simulink model "Energy2021b"  (R2021b)
settings: Solver=ode1  StartTime=0.0  StopTime=955800  FixedStep=1  RelTol=1e-3
(part 1 of 3)
settings Model: Creator=YYH  LastModifiedBy=10537
settings DebuggingCC: UnconnectedInputMsg=none  UnconnectedOutputMsg=none  UnconnectedLineMsg=none
settings ModelReferenceCC: EnableRefExpFcnMdlSchedulingChecks=off
settings RTWCC: GPUComputeCapability=5.0  DLArmComputeVersion=20.02.1

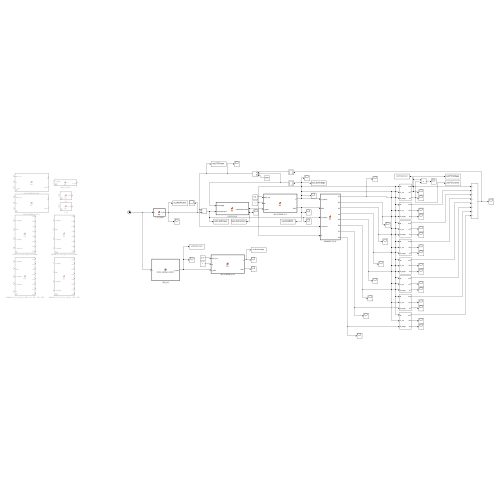
[thumbnail: Simulink's stored preview of the top-level diagram]
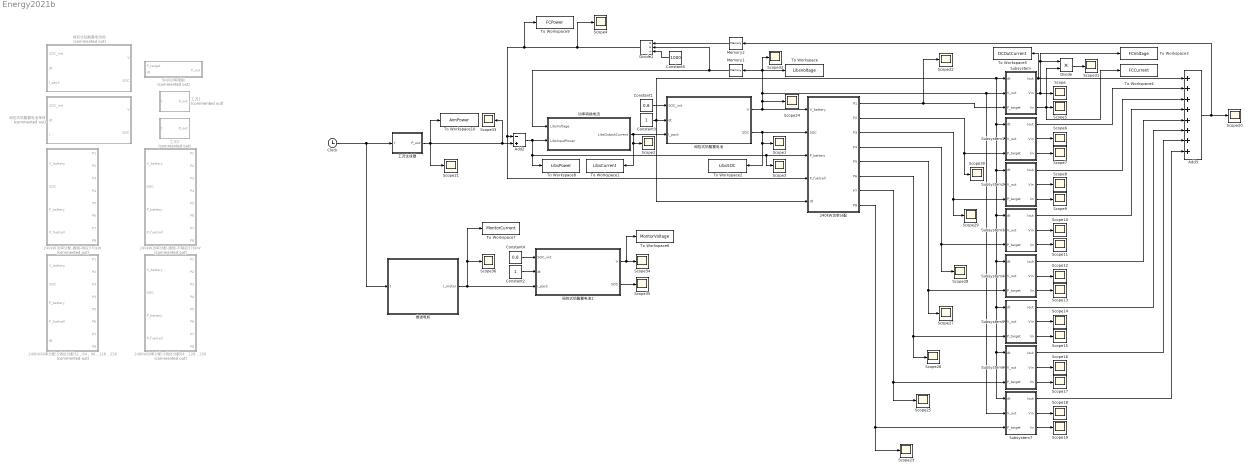
== system Energy2021b ==
  240kW功率分配 : MATLAB Function  TreatAsAtomicUnit=on
  240kW功率分配-3挡位分配64，128，256 : MATLAB Function  Commented=on  TreatAsAtomicUnit=on
  240kW功率分配-5挡位分配32，64，96，128，256 : MATLAB Function  Commented=on  TreatAsAtomicUnit=on
  240kW功率分配-跟随-不响应370kW : MATLAB Function  Commented=on  TreatAsAtomicUnit=on
  240kW功率分配-跟随-响应370kW : MATLAB Function  Commented=on  TreatAsAtomicUnit=on
  5kW功率限制 : MATLAB Function  Commented=on  TreatAsAtomicUnit=on
  Add2 : Sum  Inputs=-+
  Add3 : Sum  Inputs=++++++++
  Clock : Clock
  Constant1 : Constant  Value=0.8
  Constant2 : Constant
  Constant3 : Constant
  Constant4 : Constant  Value=0.8
  Constant5 : Constant  Value=1000
  Divide : Product  Inputs=**
  Divide1 : Product  Inputs=**/
  Memory1 : Memory  InitialCondition=487.0548
  Memory2 : Memory
  Scope{,1..36} (37 alike) : Scope
  Subsystem : Subsystem
  Subsystem1 : Subsystem
  Subsystem2 : Subsystem
  Subsystem3 : Subsystem
  Subsystem4 : Subsystem
  Subsystem5 : Subsystem
  Subsystem6 : Subsystem
  Subsystem7 : Subsystem
  To Workspace : ToWorkspace  VariableName=LibsVoltage  SaveFormat=Structure With Time  SampleTime=-1
  To Workspace1 : ToWorkspace  VariableName=LibsCurrent  SaveFormat=Structure With Time  SampleTime=-1
  To Workspace10 : ToWorkspace  VariableName=AimPower  SaveFormat=Structure With Time  SampleTime=-1
  To Workspace2 : ToWorkspace  VariableName=LibsSOC  SaveFormat=Structure With Time  SampleTime=-1
  To Workspace3 : ToWorkspace  VariableName=FCVoltage  SaveFormat=Structure With Time  SampleTime=-1
  To Workspace4 : ToWorkspace  VariableName=FCCurrent  SaveFormat=Structure With Time  SampleTime=-1
  To Workspace5 : ToWorkspace  VariableName=DCOutCurrent  SaveFormat=Structure With Time  SampleTime=-1
  To Workspace6 : ToWorkspace  VariableName=MontorVoltage  SaveFormat=Structure With Time  SampleTime=-1
  To Workspace7 : ToWorkspace  VariableName=MontorCurrent  SaveFormat=Structure With Time  SampleTime=-1
  To Workspace8 : ToWorkspace  VariableName=LibsPower  SaveFormat=Structure With Time  SampleTime=-1
  To Workspace9 : ToWorkspace  VariableName=FCPower  SaveFormat=Structure With Time  SampleTime=-1
  功率转换电流 : MATLAB Function  TreatAsAtomicUnit=on
  工况1 : MATLAB Function  Commented=on  TreatAsAtomicUnit=on
  工况2 : MATLAB Function  Commented=on  TreatAsAtomicUnit=on
  工况生成器 : MATLAB Function  TreatAsAtomicUnit=on
  推进电机 : MATLAB Function  TreatAsAtomicUnit=on
  阀控式铅酸蓄电池 : MATLAB Function  TreatAsAtomicUnit=on
  阀控式铅酸蓄电池1 : MATLAB Function  TreatAsAtomicUnit=on
  阀控式铅酸蓄电池单体 : MATLAB Function  Commented=on  TreatAsAtomicUnit=on
  阀控式铅酸蓄电池组 : MATLAB Function  Commented=on  TreatAsAtomicUnit=on
  wires:
  功率转换电流/1(LibsOutputCurrent) -> 阀控式铅酸蓄电池/3(I_pack), To Workspace1/1, Scope2/1
  Memory1/1 -> Divide1/2, 功率转换电流/1(LibsVoltage)
  阀控式铅酸蓄电池/2(SOC) -> To Workspace2/1, Scope1/1, 240kW功率分配/2(SOC)
  Constant1/1 -> 阀控式铅酸蓄电池/1(SOC_init)
  Memory2/1 -> Divide1/1
  Divide1/1 -> Scope4/1, To Workspace9/1, 240kW功率分配/4(P_fuelcell), Add2/1
  Constant5/1 -> Divide1/3
  240kW功率分配/1(P1) -> Scope22/1, Subsystem/3(P_target)
  240kW功率分配/2(P2) -> Scope30/1, Subsystem1/3(P_target)
  240kW功率分配/3(P3) -> Subsystem2/3(P_target), Scope29/1
  240kW功率分配/4(P4) -> Subsystem3/3(P_target), Scope28/1
  240kW功率分配/5(P5) -> Scope27/1, Subsystem4/3(P_target)
  240kW功率分配/8(P8) -> Subsystem7/3(P_target), Scope23/1
  240kW功率分配/7(P7) -> Subsystem6/3(P_target), Scope25/1
  Subsystem/1(Iout) -> To Workspace5/1, Add3/1
  Subsystem1/1(Iout) -> Add3/2
  Subsystem2/1(Iout) -> Add3/3
  Subsystem7/1(Iout) -> Add3/8
  Subsystem6/1(Iout) -> Add3/7
  Subsystem5/1(Iout) -> Add3/6
  Subsystem4/1(Iout) -> Add3/5
  Subsystem3/1(Iout) -> Add3/4
  Subsystem/2(Vin) -> To Workspace3/1, Divide/1, Scope/1
  Subsystem/3(Iin) -> Scope5/1, To Workspace4/1, Divide/2
  Subsystem1/3(Iin) -> Scope7/1
  Subsystem1/2(Vin) -> Scope6/1
  Subsystem2/2(Vin) -> Scope8/1
  Subsystem2/3(Iin) -> Scope9/1
  Subsystem3/2(Vin) -> Scope10/1
  Subsystem3/3(Iin) -> Scope11/1
  Subsystem4/2(Vin) -> Scope12/1
  Subsystem4/3(Iin) -> Scope13/1
  Subsystem7/3(Iin) -> Scope19/1
  Subsystem7/2(Vin) -> Scope18/1
  Subsystem6/3(Iin) -> Scope17/1
  Subsystem6/2(Vin) -> Scope16/1
  Subsystem5/3(Iin) -> Scope15/1
  Subsystem5/2(Vin) -> Scope14/1
  Add3/1 -> Memory2/1, Scope20/1
  Add2/1 -> To Workspace8/1, 240kW功率分配/3(P_battery), Scope3/1, 功率转换电流/2(LibsInputPower)
  阀控式铅酸蓄电池/1(V) -> Scope24/1, Subsystem/2(V_out), Subsystem1/2(V_out), Subsystem2/2(V_out), Subsystem3/2(V_out), Subsystem4/2(V_out), Subsystem5/2(V_out), Subsystem7/2(V_out), Subsystem6/2(V_out), Scope32/1, Memory1/1, To Workspace/1, 240kW功率分配/1(V_battery)
  240kW功率分配/6(P6) -> Subsystem5/3(P_target), Scope26/1
  Divide/1 -> Scope31/1
  Constant3/1 -> 240kW功率分配/5(dt), 阀控式铅酸蓄电池/2(dt), Subsystem1/1(dt), Subsystem2/1(dt), Subsystem3/1(dt), Subsystem4/1(dt), Subsystem5/1(dt), Subsystem7/1(dt), Subsystem6/1(dt), Subsystem/1(dt)
  Clock/1 -> 推进电机/1(t), 工况生成器/1(t)
  工况生成器/1(P_out) -> To Workspace10/1, Scope33/1, Add2/2, Scope21/1
  推进电机/1(I_motor) -> Scope36/1, To Workspace7/1, 阀控式铅酸蓄电池1/3(I_pack)
  Constant2/1 -> 阀控式铅酸蓄电池1/2(dt)
  Constant4/1 -> 阀控式铅酸蓄电池1/1(SOC_init)
  阀控式铅酸蓄电池1/1(V) -> To Workspace6/1, Scope34/1
  阀控式铅酸蓄电池1/2(SOC) -> Scope35/1

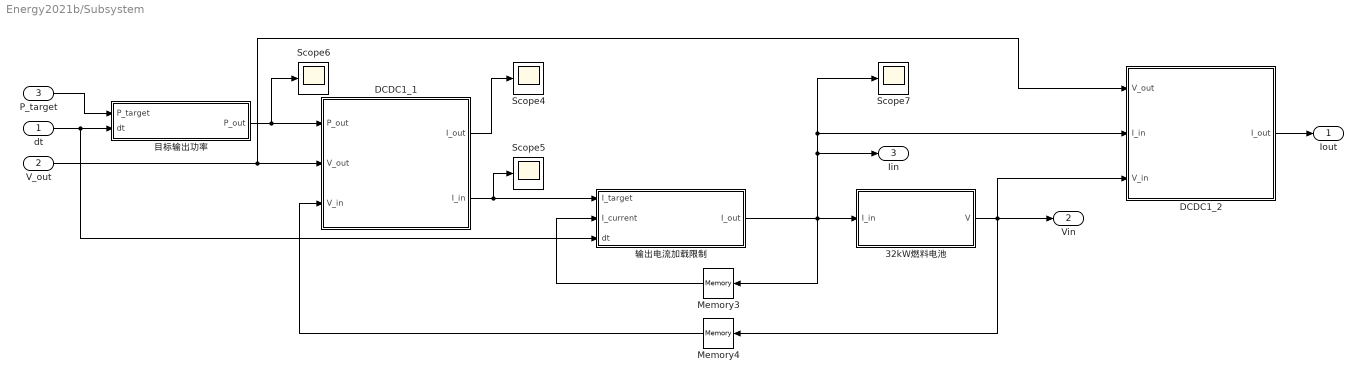
== system Energy2021b/Subsystem ==
  dt : Inport
  V_out : Inport  Port=2
  P_target : Inport  Port=3
  32kW燃料电池 : MATLAB Function  TreatAsAtomicUnit=on
  DCDC1_1 : MATLAB Function  TreatAsAtomicUnit=on
  DCDC1_2 : MATLAB Function  TreatAsAtomicUnit=on
  Memory3 : Memory
  Memory4 : Memory  InitialCondition=248.1
  Scope{4..7} (4 alike) : Scope
  目标输出功率 : MATLAB Function  TreatAsAtomicUnit=on
  输出电流加载限制 : MATLAB Function  TreatAsAtomicUnit=on
  Iout : Outport
  Vin : Outport  Port=2
  Iin : Outport  Port=3
  wires:
  dt/1 -> 输出电流加载限制/3(dt), 目标输出功率/2(dt)
  DCDC1_1/2(I_in) -> 输出电流加载限制/1(I_target), Scope5/1
  Memory4/1 -> DCDC1_1/3(V_in)
  目标输出功率/1(P_out) -> Scope6/1, DCDC1_1/1(P_out)
  32kW燃料电池/1(V) -> DCDC1_2/3(V_in), Vin/1, Memory4/1
  DCDC1_1/1(I_out) -> Scope4/1
  输出电流加载限制/1(I_out) -> Iin/1, Scope7/1, DCDC1_2/2(I_in), Memory3/1, 32kW燃料电池/1(I_in)
  Memory3/1 -> 输出电流加载限制/2(I_current)
  P_target/1 -> 目标输出功率/1(P_target)
  DCDC1_2/1(I_out) -> Iout/1
  V_out/1 -> DCDC1_2/1(V_out), DCDC1_1/2(V_out)

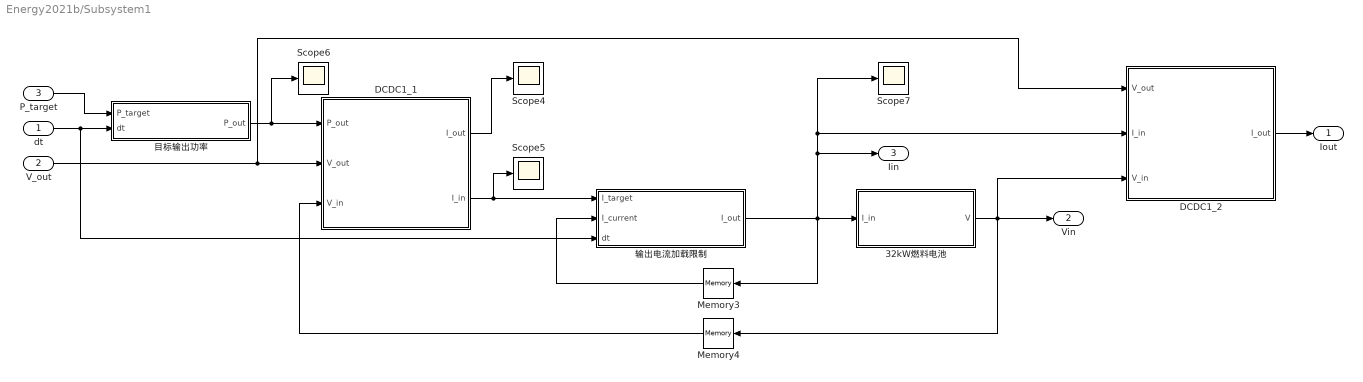
== system Energy2021b/Subsystem1 ==
  dt : Inport
  V_out : Inport  Port=2
  P_target : Inport  Port=3
  32kW燃料电池 : MATLAB Function  TreatAsAtomicUnit=on
  DCDC1_1 : MATLAB Function  TreatAsAtomicUnit=on
  DCDC1_2 : MATLAB Function  TreatAsAtomicUnit=on
  Memory3 : Memory
  Memory4 : Memory  InitialCondition=248.1
  Scope{4..7} (4 alike) : Scope
  目标输出功率 : MATLAB Function  TreatAsAtomicUnit=on
  输出电流加载限制 : MATLAB Function  TreatAsAtomicUnit=on
  Iout : Outport
  Vin : Outport  Port=2
  Iin : Outport  Port=3
  wires:
  dt/1 -> 输出电流加载限制/3(dt), 目标输出功率/2(dt)
  DCDC1_1/2(I_in) -> 输出电流加载限制/1(I_target), Scope5/1
  Memory4/1 -> DCDC1_1/3(V_in)
  目标输出功率/1(P_out) -> Scope6/1, DCDC1_1/1(P_out)
  32kW燃料电池/1(V) -> DCDC1_2/3(V_in), Vin/1, Memory4/1
  DCDC1_1/1(I_out) -> Scope4/1
  输出电流加载限制/1(I_out) -> Iin/1, Scope7/1, DCDC1_2/2(I_in), Memory3/1, 32kW燃料电池/1(I_in)
  Memory3/1 -> 输出电流加载限制/2(I_current)
  P_target/1 -> 目标输出功率/1(P_target)
  DCDC1_2/1(I_out) -> Iout/1
  V_out/1 -> DCDC1_2/1(V_out), DCDC1_1/2(V_out)

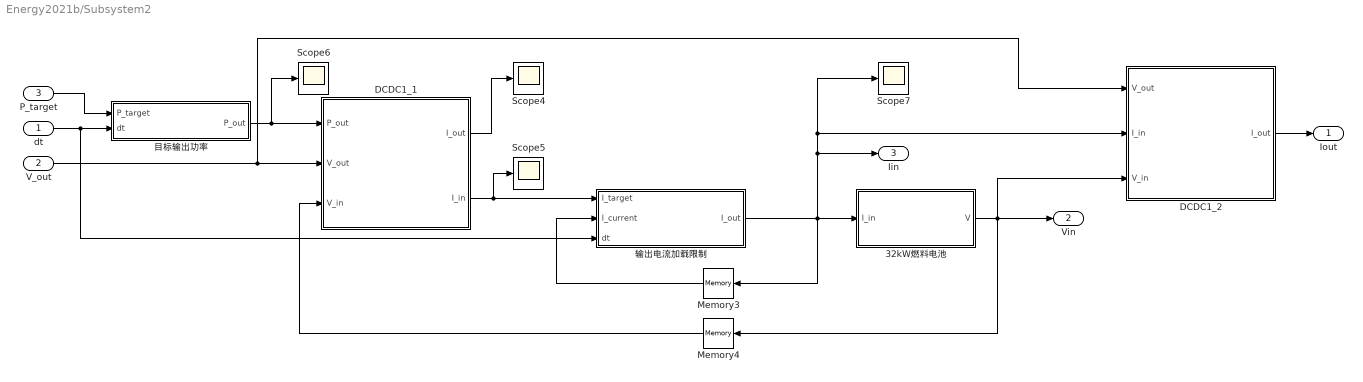
== system Energy2021b/Subsystem2 ==
  dt : Inport
  V_out : Inport  Port=2
  P_target : Inport  Port=3
  32kW燃料电池 : MATLAB Function  TreatAsAtomicUnit=on
  DCDC1_1 : MATLAB Function  TreatAsAtomicUnit=on
  DCDC1_2 : MATLAB Function  TreatAsAtomicUnit=on
  Memory3 : Memory
  Memory4 : Memory  InitialCondition=248.1
  Scope{4..7} (4 alike) : Scope
  目标输出功率 : MATLAB Function  TreatAsAtomicUnit=on
  输出电流加载限制 : MATLAB Function  TreatAsAtomicUnit=on
  Iout : Outport
  Vin : Outport  Port=2
  Iin : Outport  Port=3
  wires:
  dt/1 -> 输出电流加载限制/3(dt), 目标输出功率/2(dt)
  DCDC1_1/2(I_in) -> 输出电流加载限制/1(I_target), Scope5/1
  Memory4/1 -> DCDC1_1/3(V_in)
  目标输出功率/1(P_out) -> Scope6/1, DCDC1_1/1(P_out)
  32kW燃料电池/1(V) -> DCDC1_2/3(V_in), Vin/1, Memory4/1
  DCDC1_1/1(I_out) -> Scope4/1
  输出电流加载限制/1(I_out) -> Iin/1, Scope7/1, DCDC1_2/2(I_in), Memory3/1, 32kW燃料电池/1(I_in)
  Memory3/1 -> 输出电流加载限制/2(I_current)
  P_target/1 -> 目标输出功率/1(P_target)
  DCDC1_2/1(I_out) -> Iout/1
  V_out/1 -> DCDC1_2/1(V_out), DCDC1_1/2(V_out)

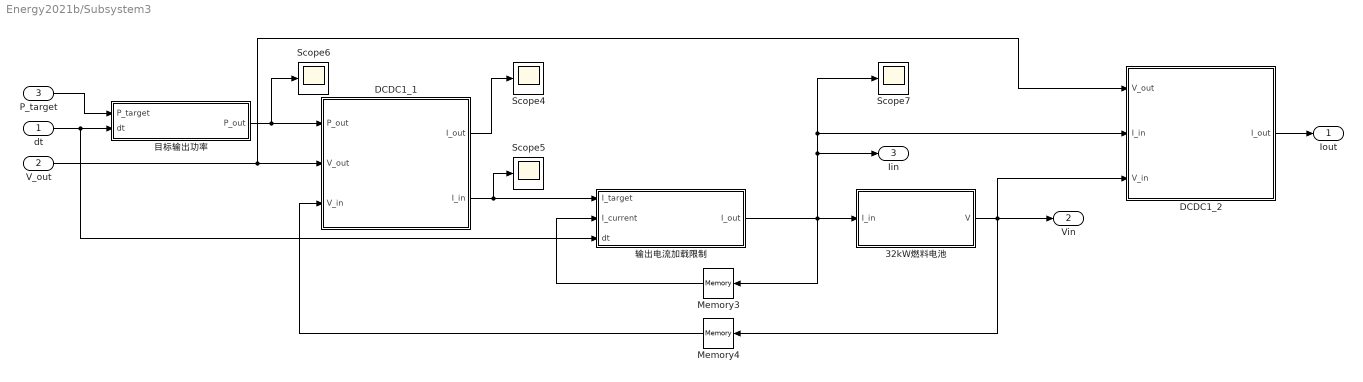
== system Energy2021b/Subsystem3 ==
  dt : Inport
  V_out : Inport  Port=2
  P_target : Inport  Port=3
  32kW燃料电池 : MATLAB Function  TreatAsAtomicUnit=on
  DCDC1_1 : MATLAB Function  TreatAsAtomicUnit=on
  DCDC1_2 : MATLAB Function  TreatAsAtomicUnit=on
  Memory3 : Memory
  Memory4 : Memory  InitialCondition=248.1
  Scope{4..7} (4 alike) : Scope
  目标输出功率 : MATLAB Function  TreatAsAtomicUnit=on
  输出电流加载限制 : MATLAB Function  TreatAsAtomicUnit=on
  Iout : Outport
  Vin : Outport  Port=2
  Iin : Outport  Port=3
  wires:
  dt/1 -> 输出电流加载限制/3(dt), 目标输出功率/2(dt)
  DCDC1_1/2(I_in) -> 输出电流加载限制/1(I_target), Scope5/1
  Memory4/1 -> DCDC1_1/3(V_in)
  目标输出功率/1(P_out) -> Scope6/1, DCDC1_1/1(P_out)
  32kW燃料电池/1(V) -> DCDC1_2/3(V_in), Vin/1, Memory4/1
  DCDC1_1/1(I_out) -> Scope4/1
  输出电流加载限制/1(I_out) -> Iin/1, Scope7/1, DCDC1_2/2(I_in), Memory3/1, 32kW燃料电池/1(I_in)
  Memory3/1 -> 输出电流加载限制/2(I_current)
  P_target/1 -> 目标输出功率/1(P_target)
  DCDC1_2/1(I_out) -> Iout/1
  V_out/1 -> DCDC1_2/1(V_out), DCDC1_1/2(V_out)

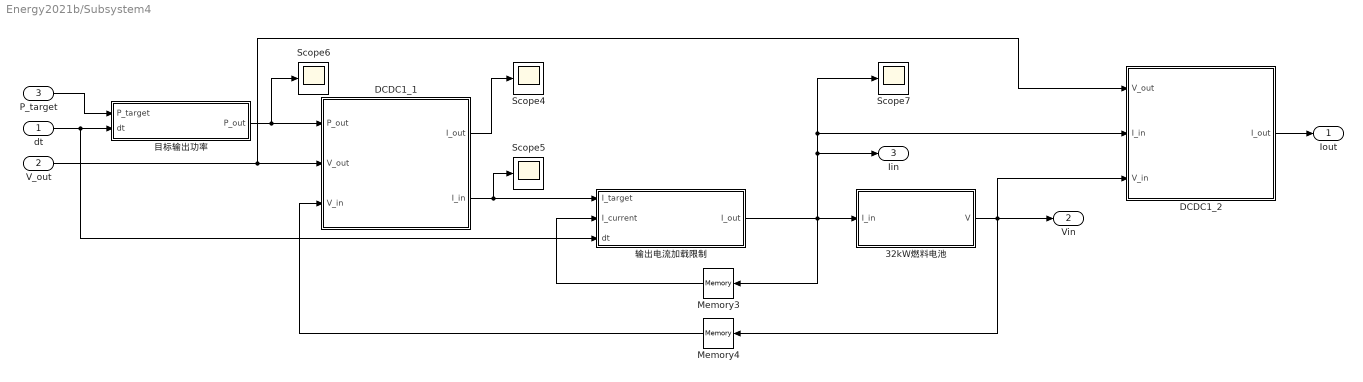
== system Energy2021b/Subsystem4 ==
  dt : Inport
  V_out : Inport  Port=2
  P_target : Inport  Port=3
  32kW燃料电池 : MATLAB Function  TreatAsAtomicUnit=on
  DCDC1_1 : MATLAB Function  TreatAsAtomicUnit=on
  DCDC1_2 : MATLAB Function  TreatAsAtomicUnit=on
  Memory3 : Memory
  Memory4 : Memory  InitialCondition=248.1
  Scope{4..7} (4 alike) : Scope
  目标输出功率 : MATLAB Function  TreatAsAtomicUnit=on
  输出电流加载限制 : MATLAB Function  TreatAsAtomicUnit=on
  Iout : Outport
  Vin : Outport  Port=2
  Iin : Outport  Port=3
  wires:
  dt/1 -> 输出电流加载限制/3(dt), 目标输出功率/2(dt)
  DCDC1_1/2(I_in) -> 输出电流加载限制/1(I_target), Scope5/1
  Memory4/1 -> DCDC1_1/3(V_in)
  目标输出功率/1(P_out) -> Scope6/1, DCDC1_1/1(P_out)
  32kW燃料电池/1(V) -> DCDC1_2/3(V_in), Vin/1, Memory4/1
  DCDC1_1/1(I_out) -> Scope4/1
  输出电流加载限制/1(I_out) -> Iin/1, Scope7/1, DCDC1_2/2(I_in), Memory3/1, 32kW燃料电池/1(I_in)
  Memory3/1 -> 输出电流加载限制/2(I_current)
  P_target/1 -> 目标输出功率/1(P_target)
  DCDC1_2/1(I_out) -> Iout/1
  V_out/1 -> DCDC1_2/1(V_out), DCDC1_1/2(V_out)

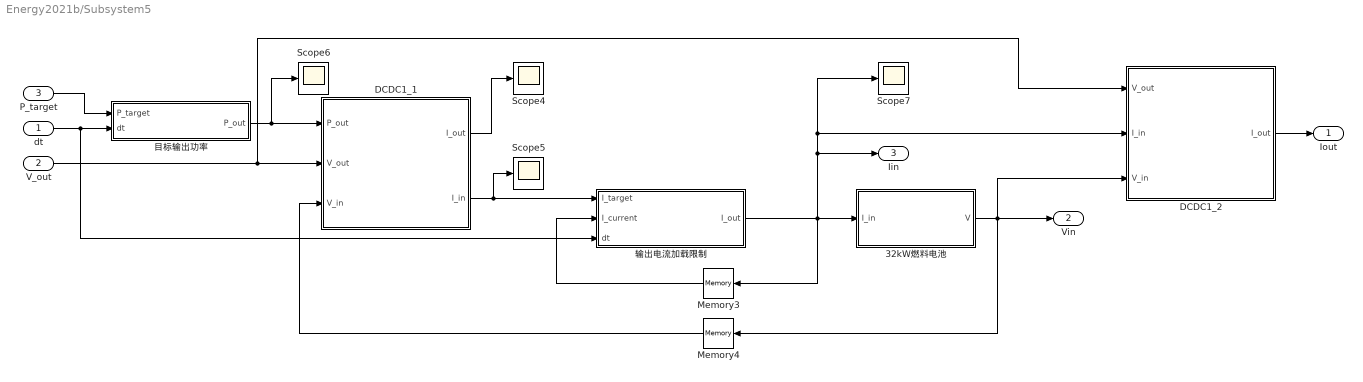
== system Energy2021b/Subsystem5 ==
  dt : Inport
  V_out : Inport  Port=2
  P_target : Inport  Port=3
  32kW燃料电池 : MATLAB Function  TreatAsAtomicUnit=on
  DCDC1_1 : MATLAB Function  TreatAsAtomicUnit=on
  DCDC1_2 : MATLAB Function  TreatAsAtomicUnit=on
  Memory3 : Memory
  Memory4 : Memory  InitialCondition=248.1
  Scope{4..7} (4 alike) : Scope
  目标输出功率 : MATLAB Function  TreatAsAtomicUnit=on
  输出电流加载限制 : MATLAB Function  TreatAsAtomicUnit=on
  Iout : Outport
  Vin : Outport  Port=2
  Iin : Outport  Port=3
  wires:
  dt/1 -> 输出电流加载限制/3(dt), 目标输出功率/2(dt)
  DCDC1_1/2(I_in) -> 输出电流加载限制/1(I_target), Scope5/1
  Memory4/1 -> DCDC1_1/3(V_in)
  目标输出功率/1(P_out) -> Scope6/1, DCDC1_1/1(P_out)
  32kW燃料电池/1(V) -> DCDC1_2/3(V_in), Vin/1, Memory4/1
  DCDC1_1/1(I_out) -> Scope4/1
  输出电流加载限制/1(I_out) -> Iin/1, Scope7/1, DCDC1_2/2(I_in), Memory3/1, 32kW燃料电池/1(I_in)
  Memory3/1 -> 输出电流加载限制/2(I_current)
  P_target/1 -> 目标输出功率/1(P_target)
  DCDC1_2/1(I_out) -> Iout/1
  V_out/1 -> DCDC1_2/1(V_out), DCDC1_1/2(V_out)

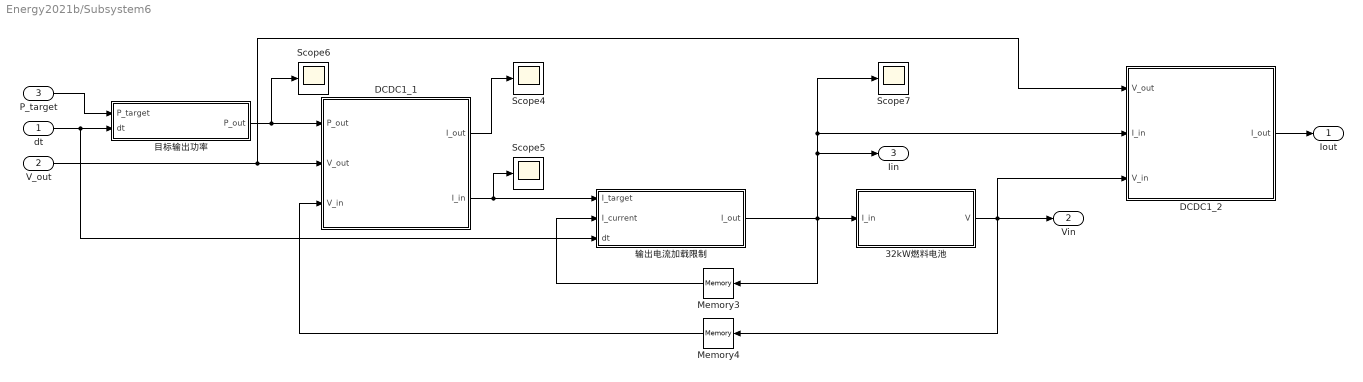
== system Energy2021b/Subsystem6 ==
  dt : Inport
  V_out : Inport  Port=2
  P_target : Inport  Port=3
  32kW燃料电池 : MATLAB Function  TreatAsAtomicUnit=on
  DCDC1_1 : MATLAB Function  TreatAsAtomicUnit=on
  DCDC1_2 : MATLAB Function  TreatAsAtomicUnit=on
  Memory3 : Memory
  Memory4 : Memory  InitialCondition=248.1
  Scope{4..7} (4 alike) : Scope
  目标输出功率 : MATLAB Function  TreatAsAtomicUnit=on
  输出电流加载限制 : MATLAB Function  TreatAsAtomicUnit=on
  Iout : Outport
  Vin : Outport  Port=2
  Iin : Outport  Port=3
  wires:
  dt/1 -> 输出电流加载限制/3(dt), 目标输出功率/2(dt)
  DCDC1_1/2(I_in) -> 输出电流加载限制/1(I_target), Scope5/1
  Memory4/1 -> DCDC1_1/3(V_in)
  目标输出功率/1(P_out) -> Scope6/1, DCDC1_1/1(P_out)
  32kW燃料电池/1(V) -> DCDC1_2/3(V_in), Vin/1, Memory4/1
  DCDC1_1/1(I_out) -> Scope4/1
  输出电流加载限制/1(I_out) -> Iin/1, Scope7/1, DCDC1_2/2(I_in), Memory3/1, 32kW燃料电池/1(I_in)
  Memory3/1 -> 输出电流加载限制/2(I_current)
  P_target/1 -> 目标输出功率/1(P_target)
  DCDC1_2/1(I_out) -> Iout/1
  V_out/1 -> DCDC1_2/1(V_out), DCDC1_1/2(V_out)

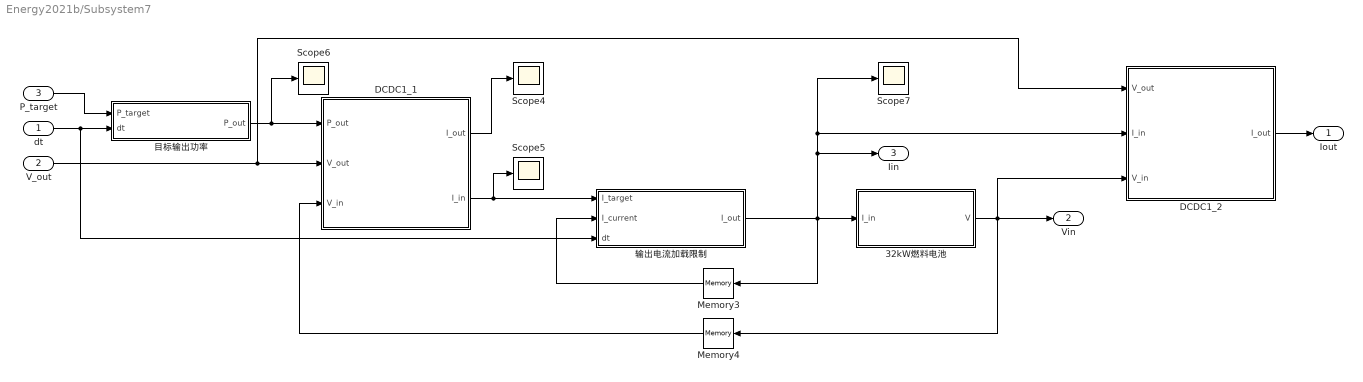
== system Energy2021b/Subsystem7 ==
  dt : Inport
  V_out : Inport  Port=2
  P_target : Inport  Port=3
  32kW燃料电池 : MATLAB Function  TreatAsAtomicUnit=on
  DCDC1_1 : MATLAB Function  TreatAsAtomicUnit=on
  DCDC1_2 : MATLAB Function  TreatAsAtomicUnit=on
  Memory3 : Memory
  Memory4 : Memory  InitialCondition=248.1
  Scope{4..7} (4 alike) : Scope
  目标输出功率 : MATLAB Function  TreatAsAtomicUnit=on
  输出电流加载限制 : MATLAB Function  TreatAsAtomicUnit=on
  Iout : Outport
  Vin : Outport  Port=2
  Iin : Outport  Port=3
  wires:
  dt/1 -> 输出电流加载限制/3(dt), 目标输出功率/2(dt)
  DCDC1_1/2(I_in) -> 输出电流加载限制/1(I_target), Scope5/1
  Memory4/1 -> DCDC1_1/3(V_in)
  目标输出功率/1(P_out) -> Scope6/1, DCDC1_1/1(P_out)
  32kW燃料电池/1(V) -> DCDC1_2/3(V_in), Vin/1, Memory4/1
  DCDC1_1/1(I_out) -> Scope4/1
  输出电流加载限制/1(I_out) -> Iin/1, Scope7/1, DCDC1_2/2(I_in), Memory3/1, 32kW燃料电池/1(I_in)
  Memory3/1 -> 输出电流加载限制/2(I_current)
  P_target/1 -> 目标输出功率/1(P_target)
  DCDC1_2/1(I_out) -> Iout/1
  V_out/1 -> DCDC1_2/1(V_out), DCDC1_1/2(V_out)

== matlab function Energy2021b/Subsystem2/目标输出功率 ==
  data: P_target input; dt input; P_out output
function P_out = fcn(P_target, dt)
%% 燃料电池预热控制器 - 带热机跳过功能
%% 输入:
%%   P_target - 目标功率 (kW)
%%   dt       - 采样时间 (s)
%% 输出:
%%   P_out    - 输出功率 (kW)

%% ===== 参数设置 =====
T_warmup = 1800;       % 预热时间 30分钟
P_warmup = 5;          % 预热功率上限 5kW
T_hot_keep = 18000;    % 热机保持时间 5小时 = 5*3600s

%% ===== 状态变量 =====
persistent timer_run timer_stop is_running is_hot
if isempty(timer_run)
    timer_run = 0;      % 运行计时器
    timer_stop = 0;     % 停机计时器
    is_running = 0;     % 运行状态
    is_hot = 0;         % 热机状态：0=冷机，1=已热机
end

%% ===== 状态机逻辑 =====
if P_target > 0
    % 启动/运行中
    if is_running == 0
        % 刚启动
        is_running = 1;
        timer_run = 0;
        
        % 判断是否需要热机
        if is_hot == 1 && timer_stop <= T_hot_keep
            % 停机5小时内，跳过热机
            timer_run = T_warmup + 1;  % 直接跳过热机阶段
        else
            % 冷机或停机超过5小时，需要热机
            timer_run = 0;
        end
    end
    
    timer_run = timer_run + dt;
    timer_stop = 0;  % 清空停机计时
    
    % 完成热机后标记
    if timer_run > T_warmup
        is_hot = 1;
    end
else
    % 停机
    if is_running == 1
        % 刚停机
        is_running = 0;
        timer_stop = 0;
    end
    
    timer_stop = timer_stop + dt;
    timer_run = 0;
    
    % 停机超过5小时，热机状态清除
    if timer_stop > T_hot_keep
        is_hot = 0;
    end
end

%% ===== 功率选择 =====
if P_target <= 0
    P_out = 0;
elseif timer_run <= T_warmup
    % 热机阶段，限制最大5kW
    P_out = min(P_target, P_warmup);
else
    % 热机完成，输出等于输入
    P_out = P_target;
end

end

== matlab function Energy2021b/Subsystem2/输出电流加载限制 ==
  data: I_target input; I_current input; I_out output; dt input
function I_out = fcn(I_target,I_current,  dt)
%% 电流斜坡控制器 - 反馈版
%% 输入:
%%   I_current - 当前电流 (A)，从输出反馈
%%   I_target  - 目标电流 (A) 
%%   dt        - 采样时间 (s)
%% 输出:
%%   I_out     - 输出电流 (A)

%% ===== 参数设置 =====
rate_up = 1;    % 上升速率 1A/s
rate_down = 2;  % 下降速率 2A/s

%% ===== 斜坡控制 =====
delta = I_target - I_current;

if delta > 0
    % 目标 > 当前，每秒+1A
    I_out = I_current + rate_up * dt;
    if I_out > I_target
        I_out = I_target;
    end
elseif delta < 0
    % 目标 < 当前，每秒-2A
    I_out = I_current - rate_down * dt;
    if I_out < I_target
        I_out = I_target;
    end
else
    I_out = I_current;
end

%% ===== 输出限幅 =====
I_out = max(0, I_out);

end

== matlab function Energy2021b/Subsystem3/32kW燃料电池 ==
  data: I_in input; V output
function V = fcn(I_in)
%% 燃料电池模型 - 极化曲线
%% 输入: I_in - 输入电流 (A)
%% 输出: V    - 输出电压 (V)

%% ===== 极化曲线数据 =====
I_table = [0, 16.77, 31.67, 48.13, 64.92, 80.76, 98.06, 115.48, 132.58, 150.51, 170.44, 186.07];
V_table = [248.1, 218.42, 212.82, 207.8, 205, 202.68, 200, 197.8, 196.44, 194.26, 192.66, 191.2];

%% ===== 电流限幅 =====
I_max = 186.07;
I = max(0, min(I_in, I_max));

%% ===== 根据电流查找电压 =====
V = V_table(1);  % 初始化
n = 12;

for k = 1:n-1
    if I >= I_table(k) && I <= I_table(k+1)
        t = (I - I_table(k)) / (I_table(k+1) - I_table(k));
        V = V_table(k) + t * (V_table(k+1) - V_table(k));
        break;
    end
end

if I >= I_table(n)
    V = V_table(n);
end

end

== matlab function Energy2021b/Subsystem3/DCDC1_1 ==
  data: P_out input; V_out input; I_out output; V_in input; I_in output
function [I_out, I_in] = fcn(P_out, V_out, V_in)
%% DCDC模型 - 输出功率反算输入电流
%% 输入:
%%   P_out - 输出功率 (W)
%%   V_out - 输出电压 (V)
%%   V_in  - 输入电压 (V)
%% 输出:
%%   I_out - 输出电流 (A)
%%   I_in  - 输入电流 (A)

%% ===== 效率MAP表 =====
% 输入电压断点 (V)
V_bp = [160, 180, 200, 220, 240, 260, 280];

% 输入电流断点 (A)
I_bp = [0, 20, 40, 60, 80, 100, 120, 140, 160, 180, 200];

% 效率表 (%)，行=电流，列=电压
Eta_map = [
    86, 86, 86, 86, 86, 86, 86;
    88, 88, 87, 87, 87, 87, 86;
    92, 91, 91, 90, 89, 88, 87;
    94, 93, 93, 92, 91, 90, 88;
    94.5, 94, 94, 93, 92, 91, 89;
    95, 94.5, 94, 93.5, 93, 91, 90;
    95, 94.5, 94.5, 94, 93, 92, 91;
    95, 95, 94.5, 94, 93.5, 93, 91;
    95, 95, 94.5, 94, 93, 92, 91;
    95, 94.5, 94.5, 93, 92, 91, 91;
    95, 94.5, 94, 92, 91, 91, 91
] / 100;

%% ===== 输出电流（直接计算） =====
V_out_safe = max(V_out, 1);
I_out = 1000*P_out / V_out_safe;

%% ===== 迭代求输入电流 =====
V_in_clamp = max(160, min(280, V_in));
V_in_safe = max(V_in, 1);

% 初始估计效率
eta = 0.94;

% 迭代3次足够收敛
for iter = 1:3
    % 根据效率计算输入功率和电流
    P_in = 1000*P_out / eta;
    I_in_est = P_in / V_in_safe;
    I_in_clamp = max(0, min(200, I_in_est));
    
    % 查表获取新效率
    eta = lookup_eta(V_in_clamp, I_in_clamp, V_bp, I_bp, Eta_map);
end

%% ===== 最终输入电流 =====
P_in = 1000*P_out / eta;
I_in = P_in / V_in_safe;

end

%% ===== 效率查表函数 =====
function eta = lookup_eta(V_in, I_in, V_bp, I_bp, Eta_map)
    % 找电压区间
    nV = 7;
    jV = 1;
    for j = 1:nV-1
        if V_in >= V_bp(j) && V_in <= V_bp(j+1)
            jV = j;
            break;
        end
    end
    if V_in >= V_bp(nV)
        jV = nV - 1;
    end
    tV = (V_in - V_bp(jV)) / (V_bp(jV+1) - V_bp(jV));
    
    % 找电流区间
    nI = 11;
    iI = 1;
    for i = 1:nI-1
        if I_in >= I_bp(i) && I_in <= I_bp(i+1)
            iI = i;
            break;
        end
    end
    if I_in >= I_bp(nI)
        iI = nI - 1;
    end
    tI = (I_in - I_bp(iI)) / (I_bp(iI+1) - I_bp(iI));
    
    % 双线性插值
    eta_11 = Eta_map(iI, jV);
    eta_12 = Eta_map(iI, jV+1);
    eta_21 = Eta_map(iI+1, jV);
    eta_22 = Eta_map(iI+1, jV+1);
    
    eta_1 = eta_11 + tV * (eta_12 - eta_11);
    eta_2 = eta_21 + tV * (eta_22 - eta_21);
    eta = eta_1 + tI * (eta_2 - eta_1);
end

== matlab function Energy2021b/Subsystem3/DCDC1_2 ==
  data: V_out input; I_in input; V_in input; I_out output
function I_out = fcn(V_out,I_in, V_in)
%% DCDC模型 - 输入电流计算输出电流
%% 输入:
%%   I_in  - 输入电流 (A)
%%   V_in  - 输入电压 (V)
%%   V_out - 输出电压 (V)
%% 输出:
%%   I_out - 输出电流 (A)

%% ===== 效率MAP表 =====
% 输入电压断点 (V)
V_bp = [160, 180, 200, 220, 240, 260, 280];

% 输入电流断点 (A)
I_bp = [0, 20, 40, 60, 80, 100, 120, 140, 160, 180, 200];

% 效率表 (%)，行=电流，列=电压
Eta_map = [
    86, 86, 86, 86, 86, 86, 86;
    88, 88, 87, 87, 87, 87, 86;
    92, 91, 91, 90, 89, 88, 87;
    94, 93, 93, 92, 91, 90, 88;
    94.5, 94, 94, 93, 92, 91, 89;
    95, 94.5, 94, 93.5, 93, 91, 90;
    95, 94.5, 94.5, 94, 93, 92, 91;
    95, 95, 94.5, 94, 93.5, 93, 91;
    95, 95, 94.5, 94, 93, 92, 91;
    95, 94.5, 94.5, 93, 92, 91, 91;
    95, 94.5, 94, 92, 91, 91, 91
] / 100;

%% ===== 输入限幅 =====
V_in_clamp = max(160, min(280, V_in));
I_in_clamp = max(0, min(200, I_in));

%% ===== 查表获取效率 =====
% 找电压区间
nV = 7;
jV = 1;
for j = 1:nV-1
    if V_in_clamp >= V_bp(j) && V_in_clamp <= V_bp(j+1)
        jV = j;
        break;
    end
end
if V_in_clamp >= V_bp(nV)
    jV = nV - 1;
end
tV = (V_in_clamp - V_bp(jV)) / (V_bp(jV+1) - V_bp(jV));

% 找电流区间
nI = 11;
iI = 1;
for i = 1:nI-1
    if I_in_clamp >= I_bp(i) && I_in_clamp <= I_bp(i+1)
        iI = i;
        break;
    end
end
if I_in_clamp >= I_bp(nI)
    iI = nI - 1;
end
tI = (I_in_clamp - I_bp(iI)) / (I_bp(iI+1) - I_bp(iI));

% 双线性插值
eta_11 = Eta_map(iI, jV);
eta_12 = Eta_map(iI, jV+1);
eta_21 = Eta_map(iI+1, jV);
eta_22 = Eta_map(iI+1, jV+1);

eta_1 = eta_11 + tV * (eta_12 - eta_11);
eta_2 = eta_21 + tV * (eta_22 - eta_21);
eta = eta_1 + tI * (eta_2 - eta_1);

%% ===== 计算输出电流 =====
P_in = V_in * I_in;
P_out = P_in * eta;
V_out_safe = max(V_out, 1);
I_out = P_out / V_out_safe;

end

== matlab function Energy2021b/Subsystem3/目标输出功率 ==
  data: P_target input; dt input; P_out output
function P_out = fcn(P_target, dt)
%% 燃料电池预热控制器 - 带热机跳过功能
%% 输入:
%%   P_target - 目标功率 (kW)
%%   dt       - 采样时间 (s)
%% 输出:
%%   P_out    - 输出功率 (kW)

%% ===== 参数设置 =====
T_warmup = 1800;       % 预热时间 30分钟
P_warmup = 5;          % 预热功率上限 5kW
T_hot_keep = 18000;    % 热机保持时间 5小时 = 5*3600s

%% ===== 状态变量 =====
persistent timer_run timer_stop is_running is_hot
if isempty(timer_run)
    timer_run = 0;      % 运行计时器
    timer_stop = 0;     % 停机计时器
    is_running = 0;     % 运行状态
    is_hot = 0;         % 热机状态：0=冷机，1=已热机
end

%% ===== 状态机逻辑 =====
if P_target > 0
    % 启动/运行中
    if is_running == 0
        % 刚启动
        is_running = 1;
        timer_run = 0;
        
        % 判断是否需要热机
        if is_hot == 1 && timer_stop <= T_hot_keep
            % 停机5小时内，跳过热机
            timer_run = T_warmup + 1;  % 直接跳过热机阶段
        else
            % 冷机或停机超过5小时，需要热机
            timer_run = 0;
        end
    end
    
    timer_run = timer_run + dt;
    timer_stop = 0;  % 清空停机计时
    
    % 完成热机后标记
    if timer_run > T_warmup
        is_hot = 1;
    end
else
    % 停机
    if is_running == 1
        % 刚停机
        is_running = 0;
        timer_stop = 0;
    end
    
    timer_stop = timer_stop + dt;
    timer_run = 0;
    
    % 停机超过5小时，热机状态清除
    if timer_stop > T_hot_keep
        is_hot = 0;
    end
end

%% ===== 功率选择 =====
if P_target <= 0
    P_out = 0;
elseif timer_run <= T_warmup
    % 热机阶段，限制最大5kW
    P_out = min(P_target, P_warmup);
else
    % 热机完成，输出等于输入
    P_out = P_target;
end

end

== matlab function Energy2021b/Subsystem3/输出电流加载限制 ==
  data: I_target input; I_current input; I_out output; dt input
function I_out = fcn(I_target,I_current,  dt)
%% 电流斜坡控制器 - 反馈版
%% 输入:
%%   I_current - 当前电流 (A)，从输出反馈
%%   I_target  - 目标电流 (A) 
%%   dt        - 采样时间 (s)
%% 输出:
%%   I_out     - 输出电流 (A)

%% ===== 参数设置 =====
rate_up = 1;    % 上升速率 1A/s
rate_down = 2;  % 下降速率 2A/s

%% ===== 斜坡控制 =====
delta = I_target - I_current;

if delta > 0
    % 目标 > 当前，每秒+1A
    I_out = I_current + rate_up * dt;
    if I_out > I_target
        I_out = I_target;
    end
elseif delta < 0
    % 目标 < 当前，每秒-2A
    I_out = I_current - rate_down * dt;
    if I_out < I_target
        I_out = I_target;
    end
else
    I_out = I_current;
end

%% ===== 输出限幅 =====
I_out = max(0, I_out);

end

== matlab function Energy2021b/Subsystem4/32kW燃料电池 ==
  data: I_in input; V output
function V = fcn(I_in)
%% 燃料电池模型 - 极化曲线
%% 输入: I_in - 输入电流 (A)
%% 输出: V    - 输出电压 (V)

%% ===== 极化曲线数据 =====
I_table = [0, 16.77, 31.67, 48.13, 64.92, 80.76, 98.06, 115.48, 132.58, 150.51, 170.44, 186.07];
V_table = [248.1, 218.42, 212.82, 207.8, 205, 202.68, 200, 197.8, 196.44, 194.26, 192.66, 191.2];

%% ===== 电流限幅 =====
I_max = 186.07;
I = max(0, min(I_in, I_max));

%% ===== 根据电流查找电压 =====
V = V_table(1);  % 初始化
n = 12;

for k = 1:n-1
    if I >= I_table(k) && I <= I_table(k+1)
        t = (I - I_table(k)) / (I_table(k+1) - I_table(k));
        V = V_table(k) + t * (V_table(k+1) - V_table(k));
        break;
    end
end

if I >= I_table(n)
    V = V_table(n);
end

end

== matlab function Energy2021b/Subsystem4/DCDC1_1 ==
  data: P_out input; V_out input; I_out output; V_in input; I_in output
function [I_out, I_in] = fcn(P_out, V_out, V_in)
%% DCDC模型 - 输出功率反算输入电流
%% 输入:
%%   P_out - 输出功率 (W)
%%   V_out - 输出电压 (V)
%%   V_in  - 输入电压 (V)
%% 输出:
%%   I_out - 输出电流 (A)
%%   I_in  - 输入电流 (A)

%% ===== 效率MAP表 =====
% 输入电压断点 (V)
V_bp = [160, 180, 200, 220, 240, 260, 280];

% 输入电流断点 (A)
I_bp = [0, 20, 40, 60, 80, 100, 120, 140, 160, 180, 200];

% 效率表 (%)，行=电流，列=电压
Eta_map = [
    86, 86, 86, 86, 86, 86, 86;
    88, 88, 87, 87, 87, 87, 86;
    92, 91, 91, 90, 89, 88, 87;
    94, 93, 93, 92, 91, 90, 88;
    94.5, 94, 94, 93, 92, 91, 89;
    95, 94.5, 94, 93.5, 93, 91, 90;
    95, 94.5, 94.5, 94, 93, 92, 91;
    95, 95, 94.5, 94, 93.5, 93, 91;
    95, 95, 94.5, 94, 93, 92, 91;
    95, 94.5, 94.5, 93, 92, 91, 91;
    95, 94.5, 94, 92, 91, 91, 91
] / 100;

%% ===== 输出电流（直接计算） =====
V_out_safe = max(V_out, 1);
I_out = 1000*P_out / V_out_safe;

%% ===== 迭代求输入电流 =====
V_in_clamp = max(160, min(280, V_in));
V_in_safe = max(V_in, 1);

% 初始估计效率
eta = 0.94;

% 迭代3次足够收敛
for iter = 1:3
    % 根据效率计算输入功率和电流
    P_in = 1000*P_out / eta;
    I_in_est = P_in / V_in_safe;
    I_in_clamp = max(0, min(200, I_in_est));
    
    % 查表获取新效率
    eta = lookup_eta(V_in_clamp, I_in_clamp, V_bp, I_bp, Eta_map);
end

%% ===== 最终输入电流 =====
P_in = 1000*P_out / eta;
I_in = P_in / V_in_safe;

end

%% ===== 效率查表函数 =====
function eta = lookup_eta(V_in, I_in, V_bp, I_bp, Eta_map)
    % 找电压区间
    nV = 7;
    jV = 1;
    for j = 1:nV-1
        if V_in >= V_bp(j) && V_in <= V_bp(j+1)
            jV = j;
            break;
        end
    end
    if V_in >= V_bp(nV)
        jV = nV - 1;
    end
    tV = (V_in - V_bp(jV)) / (V_bp(jV+1) - V_bp(jV));
    
    % 找电流区间
    nI = 11;
    iI = 1;
    for i = 1:nI-1
        if I_in >= I_bp(i) && I_in <= I_bp(i+1)
            iI = i;
            break;
        end
    end
    if I_in >= I_bp(nI)
        iI = nI - 1;
    end
    tI = (I_in - I_bp(iI)) / (I_bp(iI+1) - I_bp(iI));
    
    % 双线性插值
    eta_11 = Eta_map(iI, jV);
    eta_12 = Eta_map(iI, jV+1);
    eta_21 = Eta_map(iI+1, jV);
    eta_22 = Eta_map(iI+1, jV+1);
    
    eta_1 = eta_11 + tV * (eta_12 - eta_11);
    eta_2 = eta_21 + tV * (eta_22 - eta_21);
    eta = eta_1 + tI * (eta_2 - eta_1);
end

== matlab function Energy2021b/Subsystem4/DCDC1_2 ==
  data: V_out input; I_in input; V_in input; I_out output
function I_out = fcn(V_out,I_in, V_in)
%% DCDC模型 - 输入电流计算输出电流
%% 输入:
%%   I_in  - 输入电流 (A)
%%   V_in  - 输入电压 (V)
%%   V_out - 输出电压 (V)
%% 输出:
%%   I_out - 输出电流 (A)

%% ===== 效率MAP表 =====
% 输入电压断点 (V)
V_bp = [160, 180, 200, 220, 240, 260, 280];

% 输入电流断点 (A)
I_bp = [0, 20, 40, 60, 80, 100, 120, 140, 160, 180, 200];

% 效率表 (%)，行=电流，列=电压
Eta_map = [
    86, 86, 86, 86, 86, 86, 86;
    88, 88, 87, 87, 87, 87, 86;
    92, 91, 91, 90, 89, 88, 87;
    94, 93, 93, 92, 91, 90, 88;
    94.5, 94, 94, 93, 92, 91, 89;
    95, 94.5, 94, 93.5, 93, 91, 90;
    95, 94.5, 94.5, 94, 93, 92, 91;
    95, 95, 94.5, 94, 93.5, 93, 91;
    95, 95, 94.5, 94, 93, 92, 91;
    95, 94.5, 94.5, 93, 92, 91, 91;
    95, 94.5, 94, 92, 91, 91, 91
] / 100;

%% ===== 输入限幅 =====
V_in_clamp = max(160, min(280, V_in));
I_in_clamp = max(0, min(200, I_in));

%% ===== 查表获取效率 =====
% 找电压区间
nV = 7;
jV = 1;
for j = 1:nV-1
    if V_in_clamp >= V_bp(j) && V_in_clamp <= V_bp(j+1)
        jV = j;
        break;
    end
end
if V_in_clamp >= V_bp(nV)
    jV = nV - 1;
end
tV = (V_in_clamp - V_bp(jV)) / (V_bp(jV+1) - V_bp(jV));

% 找电流区间
nI = 11;
iI = 1;
for i = 1:nI-1
    if I_in_clamp >= I_bp(i) && I_in_clamp <= I_bp(i+1)
        iI = i;
        break;
    end
end
if I_in_clamp >= I_bp(nI)
    iI = nI - 1;
end
tI = (I_in_clamp - I_bp(iI)) / (I_bp(iI+1) - I_bp(iI));

% 双线性插值
eta_11 = Eta_map(iI, jV);
eta_12 = Eta_map(iI, jV+1);
eta_21 = Eta_map(iI+1, jV);
eta_22 = Eta_map(iI+1, jV+1);

eta_1 = eta_11 + tV * (eta_12 - eta_11);
eta_2 = eta_21 + tV * (eta_22 - eta_21);
eta = eta_1 + tI * (eta_2 - eta_1);

%% ===== 计算输出电流 =====
P_in = V_in * I_in;
P_out = P_in * eta;
V_out_safe = max(V_out, 1);
I_out = P_out / V_out_safe;

end

== matlab function Energy2021b/Subsystem1/32kW燃料电池 ==
  data: I_in input; V output
function V = fcn(I_in)
%% 燃料电池模型 - 极化曲线
%% 输入: I_in - 输入电流 (A)
%% 输出: V    - 输出电压 (V)

%% ===== 极化曲线数据 =====
I_table = [0, 16.77, 31.67, 48.13, 64.92, 80.76, 98.06, 115.48, 132.58, 150.51, 170.44, 186.07];
V_table = [248.1, 218.42, 212.82, 207.8, 205, 202.68, 200, 197.8, 196.44, 194.26, 192.66, 191.2];

%% ===== 电流限幅 =====
I_max = 186.07;
I = max(0, min(I_in, I_max));

%% ===== 根据电流查找电压 =====
V = V_table(1);  % 初始化
n = 12;

for k = 1:n-1
    if I >= I_table(k) && I <= I_table(k+1)
        t = (I - I_table(k)) / (I_table(k+1) - I_table(k));
        V = V_table(k) + t * (V_table(k+1) - V_table(k));
        break;
    end
end

if I >= I_table(n)
    V = V_table(n);
end

end

== matlab function Energy2021b/Subsystem4/目标输出功率 ==
  data: P_target input; dt input; P_out output
function P_out = fcn(P_target, dt)
%% 燃料电池预热控制器 - 带热机跳过功能
%% 输入:
%%   P_target - 目标功率 (kW)
%%   dt       - 采样时间 (s)
%% 输出:
%%   P_out    - 输出功率 (kW)

%% ===== 参数设置 =====
T_warmup = 1800;       % 预热时间 30分钟
P_warmup = 5;          % 预热功率上限 5kW
T_hot_keep = 18000;    % 热机保持时间 5小时 = 5*3600s

%% ===== 状态变量 =====
persistent timer_run timer_stop is_running is_hot
if isempty(timer_run)
    timer_run = 0;      % 运行计时器
    timer_stop = 0;     % 停机计时器
    is_running = 0;     % 运行状态
    is_hot = 0;         % 热机状态：0=冷机，1=已热机
end

%% ===== 状态机逻辑 =====
if P_target > 0
    % 启动/运行中
    if is_running == 0
        % 刚启动
        is_running = 1;
        timer_run = 0;
        
        % 判断是否需要热机
        if is_hot == 1 && timer_stop <= T_hot_keep
            % 停机5小时内，跳过热机
            timer_run = T_warmup + 1;  % 直接跳过热机阶段
        else
            % 冷机或停机超过5小时，需要热机
            timer_run = 0;
        end
    end
    
    timer_run = timer_run + dt;
    timer_stop = 0;  % 清空停机计时
    
    % 完成热机后标记
    if timer_run > T_warmup
        is_hot = 1;
    end
else
    % 停机
    if is_running == 1
        % 刚停机
        is_running = 0;
        timer_stop = 0;
    end
    
    timer_stop = timer_stop + dt;
    timer_run = 0;
    
    % 停机超过5小时，热机状态清除
    if timer_stop > T_hot_keep
        is_hot = 0;
    end
end

%% ===== 功率选择 =====
if P_target <= 0
    P_out = 0;
elseif timer_run <= T_warmup
    % 热机阶段，限制最大5kW
    P_out = min(P_target, P_warmup);
else
    % 热机完成，输出等于输入
    P_out = P_target;
end

end

== matlab function Energy2021b/Subsystem4/输出电流加载限制 ==
  data: I_target input; I_current input; I_out output; dt input
function I_out = fcn(I_target,I_current,  dt)
%% 电流斜坡控制器 - 反馈版
%% 输入:
%%   I_current - 当前电流 (A)，从输出反馈
%%   I_target  - 目标电流 (A) 
%%   dt        - 采样时间 (s)
%% 输出:
%%   I_out     - 输出电流 (A)

%% ===== 参数设置 =====
rate_up = 1;    % 上升速率 1A/s
rate_down = 2;  % 下降速率 2A/s

%% ===== 斜坡控制 =====
delta = I_target - I_current;

if delta > 0
    % 目标 > 当前，每秒+1A
    I_out = I_current + rate_up * dt;
    if I_out > I_target
        I_out = I_target;
    end
elseif delta < 0
    % 目标 < 当前，每秒-2A
    I_out = I_current - rate_down * dt;
    if I_out < I_target
        I_out = I_target;
    end
else
    I_out = I_current;
end

%% ===== 输出限幅 =====
I_out = max(0, I_out);

end

== matlab function Energy2021b/Subsystem5/32kW燃料电池 ==
  data: I_in input; V output
function V = fcn(I_in)
%% 燃料电池模型 - 极化曲线
%% 输入: I_in - 输入电流 (A)
%% 输出: V    - 输出电压 (V)

%% ===== 极化曲线数据 =====
I_table = [0, 16.77, 31.67, 48.13, 64.92, 80.76, 98.06, 115.48, 132.58, 150.51, 170.44, 186.07];
V_table = [248.1, 218.42, 212.82, 207.8, 205, 202.68, 200, 197.8, 196.44, 194.26, 192.66, 191.2];

%% ===== 电流限幅 =====
I_max = 186.07;
I = max(0, min(I_in, I_max));

%% ===== 根据电流查找电压 =====
V = V_table(1);  % 初始化
n = 12;

for k = 1:n-1
    if I >= I_table(k) && I <= I_table(k+1)
        t = (I - I_table(k)) / (I_table(k+1) - I_table(k));
        V = V_table(k) + t * (V_table(k+1) - V_table(k));
        break;
    end
end

if I >= I_table(n)
    V = V_table(n);
end

end

== matlab function Energy2021b/Subsystem5/DCDC1_1 ==
  data: P_out input; V_out input; I_out output; V_in input; I_in output
function [I_out, I_in] = fcn(P_out, V_out, V_in)
%% DCDC模型 - 输出功率反算输入电流
%% 输入:
%%   P_out - 输出功率 (W)
%%   V_out - 输出电压 (V)
%%   V_in  - 输入电压 (V)
%% 输出:
%%   I_out - 输出电流 (A)
%%   I_in  - 输入电流 (A)

%% ===== 效率MAP表 =====
% 输入电压断点 (V)
V_bp = [160, 180, 200, 220, 240, 260, 280];

% 输入电流断点 (A)
I_bp = [0, 20, 40, 60, 80, 100, 120, 140, 160, 180, 200];

% 效率表 (%)，行=电流，列=电压
Eta_map = [
    86, 86, 86, 86, 86, 86, 86;
    88, 88, 87, 87, 87, 87, 86;
    92, 91, 91, 90, 89, 88, 87;
    94, 93, 93, 92, 91, 90, 88;
    94.5, 94, 94, 93, 92, 91, 89;
    95, 94.5, 94, 93.5, 93, 91, 90;
    95, 94.5, 94.5, 94, 93, 92, 91;
    95, 95, 94.5, 94, 93.5, 93, 91;
    95, 95, 94.5, 94, 93, 92, 91;
    95, 94.5, 94.5, 93, 92, 91, 91;
    95, 94.5, 94, 92, 91, 91, 91
] / 100;

%% ===== 输出电流（直接计算） =====
V_out_safe = max(V_out, 1);
I_out = 1000*P_out / V_out_safe;

%% ===== 迭代求输入电流 =====
V_in_clamp = max(160, min(280, V_in));
V_in_safe = max(V_in, 1);

% 初始估计效率
eta = 0.94;

% 迭代3次足够收敛
for iter = 1:3
    % 根据效率计算输入功率和电流
    P_in = 1000*P_out / eta;
    I_in_est = P_in / V_in_safe;
    I_in_clamp = max(0, min(200, I_in_est));
    
    % 查表获取新效率
    eta = lookup_eta(V_in_clamp, I_in_clamp, V_bp, I_bp, Eta_map);
end

%% ===== 最终输入电流 =====
P_in = 1000*P_out / eta;
I_in = P_in / V_in_safe;

end

%% ===== 效率查表函数 =====
function eta = lookup_eta(V_in, I_in, V_bp, I_bp, Eta_map)
    % 找电压区间
    nV = 7;
    jV = 1;
    for j = 1:nV-1
        if V_in >= V_bp(j) && V_in <= V_bp(j+1)
            jV = j;
            break;
        end
    end
    if V_in >= V_bp(nV)
        jV = nV - 1;
    end
    tV = (V_in - V_bp(jV)) / (V_bp(jV+1) - V_bp(jV));
    
    % 找电流区间
    nI = 11;
    iI = 1;
    for i = 1:nI-1
        if I_in >= I_bp(i) && I_in <= I_bp(i+1)
            iI = i;
            break;
        end
    end
    if I_in >= I_bp(nI)
        iI = nI - 1;
    end
    tI = (I_in - I_bp(iI)) / (I_bp(iI+1) - I_bp(iI));
    
    % 双线性插值
    eta_11 = Eta_map(iI, jV);
    eta_12 = Eta_map(iI, jV+1);
    eta_21 = Eta_map(iI+1, jV);
    eta_22 = Eta_map(iI+1, jV+1);
    
    eta_1 = eta_11 + tV * (eta_12 - eta_11);
    eta_2 = eta_21 + tV * (eta_22 - eta_21);
    eta = eta_1 + tI * (eta_2 - eta_1);
end

== matlab function Energy2021b/Subsystem5/DCDC1_2 ==
  data: V_out input; I_in input; V_in input; I_out output
function I_out = fcn(V_out,I_in, V_in)
%% DCDC模型 - 输入电流计算输出电流
%% 输入:
%%   I_in  - 输入电流 (A)
%%   V_in  - 输入电压 (V)
%%   V_out - 输出电压 (V)
%% 输出:
%%   I_out - 输出电流 (A)

%% ===== 效率MAP表 =====
% 输入电压断点 (V)
V_bp = [160, 180, 200, 220, 240, 260, 280];

% 输入电流断点 (A)
I_bp = [0, 20, 40, 60, 80, 100, 120, 140, 160, 180, 200];

% 效率表 (%)，行=电流，列=电压
Eta_map = [
    86, 86, 86, 86, 86, 86, 86;
    88, 88, 87, 87, 87, 87, 86;
    92, 91, 91, 90, 89, 88, 87;
    94, 93, 93, 92, 91, 90, 88;
    94.5, 94, 94, 93, 92, 91, 89;
    95, 94.5, 94, 93.5, 93, 91, 90;
    95, 94.5, 94.5, 94, 93, 92, 91;
    95, 95, 94.5, 94, 93.5, 93, 91;
    95, 95, 94.5, 94, 93, 92, 91;
    95, 94.5, 94.5, 93, 92, 91, 91;
    95, 94.5, 94, 92, 91, 91, 91
] / 100;

%% ===== 输入限幅 =====
V_in_clamp = max(160, min(280, V_in));
I_in_clamp = max(0, min(200, I_in));

%% ===== 查表获取效率 =====
% 找电压区间
nV = 7;
jV = 1;
for j = 1:nV-1
    if V_in_clamp >= V_bp(j) && V_in_clamp <= V_bp(j+1)
        jV = j;
        break;
    end
end
if V_in_clamp >= V_bp(nV)
    jV = nV - 1;
end
tV = (V_in_clamp - V_bp(jV)) / (V_bp(jV+1) - V_bp(jV));

% 找电流区间
nI = 11;
iI = 1;
for i = 1:nI-1
    if I_in_clamp >= I_bp(i) && I_in_clamp <= I_bp(i+1)
        iI = i;
        break;
    end
end
if I_in_clamp >= I_bp(nI)
    iI = nI - 1;
end
tI = (I_in_clamp - I_bp(iI)) / (I_bp(iI+1) - I_bp(iI));

% 双线性插值
eta_11 = Eta_map(iI, jV);
eta_12 = Eta_map(iI, jV+1);
eta_21 = Eta_map(iI+1, jV);
eta_22 = Eta_map(iI+1, jV+1);

eta_1 = eta_11 + tV * (eta_12 - eta_11);
eta_2 = eta_21 + tV * (eta_22 - eta_21);
eta = eta_1 + tI * (eta_2 - eta_1);

%% ===== 计算输出电流 =====
P_in = V_in * I_in;
P_out = P_in * eta;
V_out_safe = max(V_out, 1);
I_out = P_out / V_out_safe;

end

== matlab function Energy2021b/Subsystem5/目标输出功率 ==
  data: P_target input; dt input; P_out output
function P_out = fcn(P_target, dt)
%% 燃料电池预热控制器 - 带热机跳过功能
%% 输入:
%%   P_target - 目标功率 (kW)
%%   dt       - 采样时间 (s)
%% 输出:
%%   P_out    - 输出功率 (kW)

%% ===== 参数设置 =====
T_warmup = 1800;       % 预热时间 30分钟
P_warmup = 5;          % 预热功率上限 5kW
T_hot_keep = 18000;    % 热机保持时间 5小时 = 5*3600s

%% ===== 状态变量 =====
persistent timer_run timer_stop is_running is_hot
if isempty(timer_run)
    timer_run = 0;      % 运行计时器
    timer_stop = 0;     % 停机计时器
    is_running = 0;     % 运行状态
    is_hot = 0;         % 热机状态：0=冷机，1=已热机
end

%% ===== 状态机逻辑 =====
if P_target > 0
    % 启动/运行中
    if is_running == 0
        % 刚启动
        is_running = 1;
        timer_run = 0;
        
        % 判断是否需要热机
        if is_hot == 1 && timer_stop <= T_hot_keep
            % 停机5小时内，跳过热机
            timer_run = T_warmup + 1;  % 直接跳过热机阶段
        else
            % 冷机或停机超过5小时，需要热机
            timer_run = 0;
        end
    end
    
    timer_run = timer_run + dt;
    timer_stop = 0;  % 清空停机计时
    
    % 完成热机后标记
    if timer_run > T_warmup
        is_hot = 1;
    end
else
    % 停机
    if is_running == 1
        % 刚停机
        is_running = 0;
        timer_stop = 0;
    end
    
    timer_stop = timer_stop + dt;
    timer_run = 0;
    
    % 停机超过5小时，热机状态清除
    if timer_stop > T_hot_keep
        is_hot = 0;
    end
end

%% ===== 功率选择 =====
if P_target <= 0
    P_out = 0;
elseif timer_run <= T_warmup
    % 热机阶段，限制最大5kW
    P_out = min(P_target, P_warmup);
else
    % 热机完成，输出等于输入
    P_out = P_target;
end

end

== matlab function Energy2021b/Subsystem5/输出电流加载限制 ==
  data: I_target input; I_current input; I_out output; dt input
function I_out = fcn(I_target,I_current,  dt)
%% 电流斜坡控制器 - 反馈版
%% 输入:
%%   I_current - 当前电流 (A)，从输出反馈
%%   I_target  - 目标电流 (A) 
%%   dt        - 采样时间 (s)
%% 输出:
%%   I_out     - 输出电流 (A)

%% ===== 参数设置 =====
rate_up = 1;    % 上升速率 1A/s
rate_down = 2;  % 下降速率 2A/s

%% ===== 斜坡控制 =====
delta = I_target - I_current;

if delta > 0
    % 目标 > 当前，每秒+1A
    I_out = I_current + rate_up * dt;
    if I_out > I_target
        I_out = I_target;
    end
elseif delta < 0
    % 目标 < 当前，每秒-2A
    I_out = I_current - rate_down * dt;
    if I_out < I_target
        I_out = I_target;
    end
else
    I_out = I_current;
end

%% ===== 输出限幅 =====
I_out = max(0, I_out);

end

== matlab function Energy2021b/Subsystem6/32kW燃料电池 ==
  data: I_in input; V output
function V = fcn(I_in)
%% 燃料电池模型 - 极化曲线
%% 输入: I_in - 输入电流 (A)
%% 输出: V    - 输出电压 (V)

%% ===== 极化曲线数据 =====
I_table = [0, 16.77, 31.67, 48.13, 64.92, 80.76, 98.06, 115.48, 132.58, 150.51, 170.44, 186.07];
V_table = [248.1, 218.42, 212.82, 207.8, 205, 202.68, 200, 197.8, 196.44, 194.26, 192.66, 191.2];

%% ===== 电流限幅 =====
I_max = 186.07;
I = max(0, min(I_in, I_max));

%% ===== 根据电流查找电压 =====
V = V_table(1);  % 初始化
n = 12;

for k = 1:n-1
    if I >= I_table(k) && I <= I_table(k+1)
        t = (I - I_table(k)) / (I_table(k+1) - I_table(k));
        V = V_table(k) + t * (V_table(k+1) - V_table(k));
        break;
    end
end

if I >= I_table(n)
    V = V_table(n);
end

end

== matlab function Energy2021b/Subsystem6/DCDC1_1 ==
  data: P_out input; V_out input; I_out output; V_in input; I_in output
function [I_out, I_in] = fcn(P_out, V_out, V_in)
%% DCDC模型 - 输出功率反算输入电流
%% 输入:
%%   P_out - 输出功率 (W)
%%   V_out - 输出电压 (V)
%%   V_in  - 输入电压 (V)
%% 输出:
%%   I_out - 输出电流 (A)
%%   I_in  - 输入电流 (A)

%% ===== 效率MAP表 =====
% 输入电压断点 (V)
V_bp = [160, 180, 200, 220, 240, 260, 280];

% 输入电流断点 (A)
I_bp = [0, 20, 40, 60, 80, 100, 120, 140, 160, 180, 200];

% 效率表 (%)，行=电流，列=电压
Eta_map = [
    86, 86, 86, 86, 86, 86, 86;
    88, 88, 87, 87, 87, 87, 86;
    92, 91, 91, 90, 89, 88, 87;
    94, 93, 93, 92, 91, 90, 88;
    94.5, 94, 94, 93, 92, 91, 89;
    95, 94.5, 94, 93.5, 93, 91, 90;
    95, 94.5, 94.5, 94, 93, 92, 91;
    95, 95, 94.5, 94, 93.5, 93, 91;
    95, 95, 94.5, 94, 93, 92, 91;
    95, 94.5, 94.5, 93, 92, 91, 91;
    95, 94.5, 94, 92, 91, 91, 91
] / 100;

%% ===== 输出电流（直接计算） =====
V_out_safe = max(V_out, 1);
I_out = 1000*P_out / V_out_safe;

%% ===== 迭代求输入电流 =====
V_in_clamp = max(160, min(280, V_in));
V_in_safe = max(V_in, 1);

% 初始估计效率
eta = 0.94;

% 迭代3次足够收敛
for iter = 1:3
    % 根据效率计算输入功率和电流
    P_in = 1000*P_out / eta;
    I_in_est = P_in / V_in_safe;
    I_in_clamp = max(0, min(200, I_in_est));
    
    % 查表获取新效率
    eta = lookup_eta(V_in_clamp, I_in_clamp, V_bp, I_bp, Eta_map);
end

%% ===== 最终输入电流 =====
P_in = 1000*P_out / eta;
I_in = P_in / V_in_safe;

end

%% ===== 效率查表函数 =====
function eta = lookup_eta(V_in, I_in, V_bp, I_bp, Eta_map)
    % 找电压区间
    nV = 7;
    jV = 1;
    for j = 1:nV-1
        if V_in >= V_bp(j) && V_in <= V_bp(j+1)
            jV = j;
            break;
        end
    end
    if V_in >= V_bp(nV)
        jV = nV - 1;
    end
    tV = (V_in - V_bp(jV)) / (V_bp(jV+1) - V_bp(jV));
    
    % 找电流区间
    nI = 11;
    iI = 1;
    for i = 1:nI-1
        if I_in >= I_bp(i) && I_in <= I_bp(i+1)
            iI = i;
            break;
        end
    end
    if I_in >= I_bp(nI)
        iI = nI - 1;
    end
    tI = (I_in - I_bp(iI)) / (I_bp(iI+1) - I_bp(iI));
    
    % 双线性插值
    eta_11 = Eta_map(iI, jV);
    eta_12 = Eta_map(iI, jV+1);
    eta_21 = Eta_map(iI+1, jV);
    eta_22 = Eta_map(iI+1, jV+1);
    
    eta_1 = eta_11 + tV * (eta_12 - eta_11);
    eta_2 = eta_21 + tV * (eta_22 - eta_21);
    eta = eta_1 + tI * (eta_2 - eta_1);
end

== matlab function Energy2021b/Subsystem1/DCDC1_1 ==
  data: P_out input; V_out input; I_out output; V_in input; I_in output
function [I_out, I_in] = fcn(P_out, V_out, V_in)
%% DCDC模型 - 输出功率反算输入电流
%% 输入:
%%   P_out - 输出功率 (W)
%%   V_out - 输出电压 (V)
%%   V_in  - 输入电压 (V)
%% 输出:
%%   I_out - 输出电流 (A)
%%   I_in  - 输入电流 (A)

%% ===== 效率MAP表 =====
% 输入电压断点 (V)
V_bp = [160, 180, 200, 220, 240, 260, 280];

% 输入电流断点 (A)
I_bp = [0, 20, 40, 60, 80, 100, 120, 140, 160, 180, 200];

% 效率表 (%)，行=电流，列=电压
Eta_map = [
    86, 86, 86, 86, 86, 86, 86;
    88, 88, 87, 87, 87, 87, 86;
    92, 91, 91, 90, 89, 88, 87;
    94, 93, 93, 92, 91, 90, 88;
    94.5, 94, 94, 93, 92, 91, 89;
    95, 94.5, 94, 93.5, 93, 91, 90;
    95, 94.5, 94.5, 94, 93, 92, 91;
    95, 95, 94.5, 94, 93.5, 93, 91;
    95, 95, 94.5, 94, 93, 92, 91;
    95, 94.5, 94.5, 93, 92, 91, 91;
    95, 94.5, 94, 92, 91, 91, 91
] / 100;

%% ===== 输出电流（直接计算） =====
V_out_safe = max(V_out, 1);
I_out = 1000*P_out / V_out_safe;

%% ===== 迭代求输入电流 =====
V_in_clamp = max(160, min(280, V_in));
V_in_safe = max(V_in, 1);

% 初始估计效率
eta = 0.94;

% 迭代3次足够收敛
for iter = 1:3
    % 根据效率计算输入功率和电流
    P_in = 1000*P_out / eta;
    I_in_est = P_in / V_in_safe;
    I_in_clamp = max(0, min(200, I_in_est));
    
    % 查表获取新效率
    eta = lookup_eta(V_in_clamp, I_in_clamp, V_bp, I_bp, Eta_map);
end

%% ===== 最终输入电流 =====
P_in = 1000*P_out / eta;
I_in = P_in / V_in_safe;

end

%% ===== 效率查表函数 =====
function eta = lookup_eta(V_in, I_in, V_bp, I_bp, Eta_map)
    % 找电压区间
    nV = 7;
    jV = 1;
    for j = 1:nV-1
        if V_in >= V_bp(j) && V_in <= V_bp(j+1)
            jV = j;
            break;
        end
    end
    if V_in >= V_bp(nV)
        jV = nV - 1;
    end
    tV = (V_in - V_bp(jV)) / (V_bp(jV+1) - V_bp(jV));
    
    % 找电流区间
    nI = 11;
    iI = 1;
    for i = 1:nI-1
        if I_in >= I_bp(i) && I_in <= I_bp(i+1)
            iI = i;
            break;
        end
    end
    if I_in >= I_bp(nI)
        iI = nI - 1;
    end
    tI = (I_in - I_bp(iI)) / (I_bp(iI+1) - I_bp(iI));
    
    % 双线性插值
    eta_11 = Eta_map(iI, jV);
    eta_12 = Eta_map(iI, jV+1);
    eta_21 = Eta_map(iI+1, jV);
    eta_22 = Eta_map(iI+1, jV+1);
    
    eta_1 = eta_11 + tV * (eta_12 - eta_11);
    eta_2 = eta_21 + tV * (eta_22 - eta_21);
    eta = eta_1 + tI * (eta_2 - eta_1);
end

== matlab function Energy2021b/功率转换电流 ==
  data: LibsVoltage input; LibsInputPower input; LibsOutputCurrent output
function LibsOutputCurrent = fcn(LibsVoltage,LibsInputPower)

LibsOutputCurrent=1000*LibsInputPower/LibsVoltage;

== matlab function Energy2021b/阀控式铅酸蓄电池 ==
  data: SOC_init input; dt input; V output; I_pack input; SOC output
function [V, SOC] = fcn(SOC_init,dt,I_pack)
%% VRLA电池组二阶RC模型 - 231串2并
%% 输入: I_pack - 电池组电流(A), 放电为正
%% 输出: V - 电池组电压(V), SOC - 荷电状态(0~1)

%% ===== 电池组配置 =====
N_series = 231;    % 串联数量
N_parallel = 2;    % 并联数量

%% ===== 单体参数 =====
Q_10h = 1025.0000;
k_peukert = 1.273470;
SOC_bp = [1.00, 0.90, 0.80, 0.70, 0.60, 0.50, 0.40, 0.30, 0.20, 0.10, 0.05, 0.00];
OCV_table = [2.1500, 2.1271, 2.1077, 2.0929, 2.0783, 2.0600, 2.0384, 2.0107, 1.9800, 1.9502, 1.9352, 1.9200];
R0_table = [0.000258, 0.000258, 0.000258, 0.000258, 0.000258, 0.000258, 0.000258, 0.000258, 0.000258, 0.000260, 0.000262, 0.000268];
R1_table = [0.000020, 0.000020, 0.000020, 0.000020, 0.000020, 0.000020, 0.000020, 0.000022, 0.000030, 0.000065, 0.000114, 0.000220];
R2_table = [0.000080, 0.000080, 0.000080, 0.000080, 0.000080, 0.000080, 0.000082, 0.000089, 0.000120, 0.000259, 0.000458, 0.000880];
tau1 = 150.0000;
tau2 = 1250.0889;
alpha = 0.300000;

%% ===== 并联分流：计算单体电流 =====
I = I_pack / N_parallel;

%% ===== 模型计算(勿改) =====
persistent SOC_s V1 V2 flag
if isempty(flag), SOC_s=SOC_init; V1=0; V2=0; flag=1; end
s = max(0.001, min(1, SOC_s));
Ia = max(abs(I), 0.1);
Qe = Q_10h * (100/Ia)^(k_peukert-1);

%% 初始化变量
OCV = OCV_table(1); R0 = R0_table(1); R1b = R1_table(1); R2b = R2_table(1);

%% 线性插值
n = 12;
for k=1:n-1
    if s<=SOC_bp(k) && s>=SOC_bp(k+1)
        t=(s-SOC_bp(k+1))/(SOC_bp(k)-SOC_bp(k+1));
        OCV=OCV_table(k+1)+t*(OCV_table(k)-OCV_table(k+1));
        R0=R0_table(k+1)+t*(R0_table(k)-R0_table(k+1));
        R1b=R1_table(k+1)+t*(R1_table(k)-R1_table(k+1));
        R2b=R2_table(k+1)+t*(R2_table(k)-R2_table(k+1));
        break;
    end
end

If = (Ia/100)^(alpha-1);
R1 = R1b*If; R2 = R2b*If;
e1=exp(-dt/tau1); e2=exp(-dt/tau2);
V1=V1*e1+I*R1*(1-e1);
V2=V2*e2+I*R2*(1-e2);

%% ===== 单体电压 =====
V_cell = OCV - I*R0 - V1 - V2;
V_cell = max(1.6, min(2.4, V_cell));

%% ===== 串联：电池组电压 =====
V = N_series * V_cell;

%% ===== SOC更新 =====
SOC_s = max(0, min(1, s - I*dt/(3600*Qe)));
SOC = SOC_s;
end

== matlab function Energy2021b/阀控式铅酸蓄电池组 ==
  data: SOC_init input; dt input; V output; I_pack input; SOC output
function [V, SOC] = fcn(SOC_init,dt,I_pack)
%% VRLA电池组二阶RC模型 - 231串2并
%% 输入: I_pack - 电池组电流(A), 放电为正
%% 输出: V - 电池组电压(V), SOC - 荷电状态(0~1)

%% ===== 电池组配置 =====
N_series = 231;    % 串联数量
N_parallel = 2;    % 并联数量

%% ===== 单体参数 =====
Q_10h = 1025.0000;
k_peukert = 1.273470;
SOC_bp = [1.00, 0.90, 0.80, 0.70, 0.60, 0.50, 0.40, 0.30, 0.20, 0.10, 0.05, 0.00];
OCV_table = [2.1500, 2.1271, 2.1077, 2.0929, 2.0783, 2.0600, 2.0384, 2.0107, 1.9800, 1.9502, 1.9352, 1.9200];
R0_table = [0.000258, 0.000258, 0.000258, 0.000258, 0.000258, 0.000258, 0.000258, 0.000258, 0.000258, 0.000260, 0.000262, 0.000268];
R1_table = [0.000020, 0.000020, 0.000020, 0.000020, 0.000020, 0.000020, 0.000020, 0.000022, 0.000030, 0.000065, 0.000114, 0.000220];
R2_table = [0.000080, 0.000080, 0.000080, 0.000080, 0.000080, 0.000080, 0.000082, 0.000089, 0.000120, 0.000259, 0.000458, 0.000880];
tau1 = 150.0000;
tau2 = 1250.0889;
alpha = 0.300000;

%% ===== 并联分流：计算单体电流 =====
I = I_pack / N_parallel;

%% ===== 模型计算(勿改) =====
persistent SOC_s V1 V2 flag
if isempty(flag), SOC_s=SOC_init; V1=0; V2=0; flag=1; end
s = max(0.001, min(1, SOC_s));
Ia = max(abs(I), 0.1);
Qe = Q_10h * (100/Ia)^(k_peukert-1);

%% 初始化变量
OCV = OCV_table(1); R0 = R0_table(1); R1b = R1_table(1); R2b = R2_table(1);

%% 线性插值
n = 12;
for k=1:n-1
    if s<=SOC_bp(k) && s>=SOC_bp(k+1)
        t=(s-SOC_bp(k+1))/(SOC_bp(k)-SOC_bp(k+1));
        OCV=OCV_table(k+1)+t*(OCV_table(k)-OCV_table(k+1));
        R0=R0_table(k+1)+t*(R0_table(k)-R0_table(k+1));
        R1b=R1_table(k+1)+t*(R1_table(k)-R1_table(k+1));
        R2b=R2_table(k+1)+t*(R2_table(k)-R2_table(k+1));
        break;
    end
end

If = (Ia/100)^(alpha-1);
R1 = R1b*If; R2 = R2b*If;
e1=exp(-dt/tau1); e2=exp(-dt/tau2);
V1=V1*e1+I*R1*(1-e1);
V2=V2*e2+I*R2*(1-e2);

%% ===== 单体电压 =====
V_cell = OCV - I*R0 - V1 - V2;
V_cell = max(1.6, min(2.4, V_cell));

%% ===== 串联：电池组电压 =====
V = N_series * V_cell;

%% ===== SOC更新 =====
SOC_s = max(0, min(1, s - I*dt/(3600*Qe)));
SOC = SOC_s;
end
